simulink model "OFDM_Tx_Rx_fixed_point"  (R2020a)
settings: Solver=FixedStepDiscrete  StartTime=0.0  StopTime=inf  RelTol=1e-3
PostLoadFcn:
  | filter_setup;
InitFcn:
  | % Set parameters
  | fs = 1e6;
  | 
  | % Load all required variables
  | load('read_addr_data');
  | load('read_addr_cp');
  | load('read_addr_pream');
  | load('read_addr_rx');
  | load('pilot');
  | load('sc_index');
  | load('LTSfreq');
  | load('STSfreq');
  | load('LTSread');
  | load('STSread');
values from neighbouring files (symbols this model uses):
  CIC_fine_Rx = 2^(-(CIC_right_shift_Rx-CIC_shift_Rx))    [filter_setup.m]
  CIC_fine_Tx = 2^-(CIC_right_shift - CIC_left_shift - CIC_shift_Tx)    [filter_setup.m]
  STSfreq = [0 0 0 0 0 0 0 0 1 0 0 0 ... (64 elements, 1x64)]    [STSfreq.mat]
undefined symbols (not defined in the file or in its folder): LTSfreq, LTSread, pilot, read_addr_cp, read_addr_data, read_addr_pream, read_addr_rx, sc_index, STSread
libraries: hdlsllib x56, simulink x55, dspmlti4 x8, commseqgen3 x7, dsphdlmathfun x3, dsphdlxfrm x2, dspobslib x1, dsphdlsigops x1
(part 4 of 4)

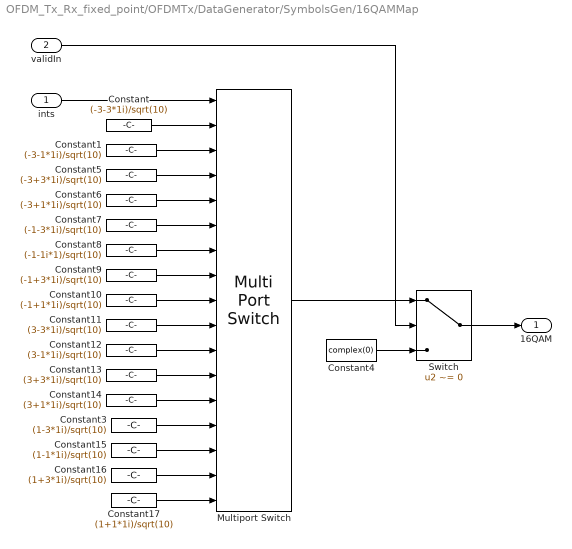
== system OFDM_Tx_Rx_fixed_point/OFDMTx/DataGenerator/SymbolsGen/16QAMMap ==
  ints : Inport
  validIn : Inport  Port=2
  Constant : Constant  Value=(-3-3*1i)/sqrt(10)  VectorParams1D=off  OutDataTypeStr=fixdt(1,16,14)  SampleTime=1/fs
  Constant1 : Constant  Value=(-3-1*1i)/sqrt(10)  VectorParams1D=off  OutDataTypeStr=fixdt(1,16,14)  SampleTime=1/fs
  Constant10 : Constant  Value=(-1+1*1i)/sqrt(10)  VectorParams1D=off  OutDataTypeStr=fixdt(1,16,14)  SampleTime=1/fs
  Constant11 : Constant  Value=(3-3*1i)/sqrt(10)  VectorParams1D=off  OutDataTypeStr=fixdt(1,16,14)  SampleTime=1/fs
  Constant12 : Constant  Value=(3-1*1i)/sqrt(10)  VectorParams1D=off  OutDataTypeStr=fixdt(1,16,14)  SampleTime=1/fs
  Constant13 : Constant  Value=(3+3*1i)/sqrt(10)  VectorParams1D=off  OutDataTypeStr=fixdt(1,16,14)  SampleTime=1/fs
  Constant14 : Constant  Value=(3+1*1i)/sqrt(10)  VectorParams1D=off  OutDataTypeStr=fixdt(1,16,14)  SampleTime=1/fs
  Constant15 : Constant  Value=(1-1*1i)/sqrt(10)  VectorParams1D=off  OutDataTypeStr=fixdt(1,16,14)  SampleTime=1/fs
  Constant16 : Constant  Value=(1+3*1i)/sqrt(10)  VectorParams1D=off  OutDataTypeStr=fixdt(1,16,14)  SampleTime=1/fs
  Constant17 : Constant  Value=(1+1*1i)/sqrt(10)  VectorParams1D=off  OutDataTypeStr=fixdt(1,16,14)  SampleTime=1/fs
  Constant3 : Constant  Value=(1-3*1i)/sqrt(10)  VectorParams1D=off  OutDataTypeStr=fixdt(1,16,14)  SampleTime=1/fs
  Constant4 : Constant  Value=complex(0)  VectorParams1D=off  OutDataTypeStr=fixdt(1,16,14)  SampleTime=1/fs
  Constant5 : Constant  Value=(-3+3*1i)/sqrt(10)  VectorParams1D=off  OutDataTypeStr=fixdt(1,16,14)  SampleTime=1/fs
  Constant6 : Constant  Value=(-3+1*1i)/sqrt(10)  VectorParams1D=off  OutDataTypeStr=fixdt(1,16,14)  SampleTime=1/fs
  Constant7 : Constant  Value=(-1-3*1i)/sqrt(10)  VectorParams1D=off  OutDataTypeStr=fixdt(1,16,14)  SampleTime=1/fs
  Constant8 : Constant  Value=(-1-1i*1)/sqrt(10)  VectorParams1D=off  OutDataTypeStr=fixdt(1,16,14)  SampleTime=1/fs
  Constant9 : Constant  Value=(-1+3*1i)/sqrt(10)  VectorParams1D=off  OutDataTypeStr=fixdt(1,16,14)  SampleTime=1/fs
  Multiport Switch : MultiPortSwitch  DataPortOrder=Zero-based contiguous  Inputs=16  zeroidx=on
  Switch : Switch  Criteria=u2 ~= 0
  16QAM : Outport  VectorParamsAs1DForOutWhenUnconnected=off
  wires:
  Switch/1 -> 16QAM/1
  Constant4/1 -> Switch/3
  Multiport Switch/1 -> Switch/1
  validIn/1 -> Switch/2
  ints/1 -> Multiport Switch/1
  Constant/1 -> Multiport Switch/2
  Constant1/1 -> Multiport Switch/3
  Constant5/1 -> Multiport Switch/4
  Constant6/1 -> Multiport Switch/5
  Constant7/1 -> Multiport Switch/6
  Constant8/1 -> Multiport Switch/7
  Constant9/1 -> Multiport Switch/8
  Constant10/1 -> Multiport Switch/9
  Constant11/1 -> Multiport Switch/10
  Constant12/1 -> Multiport Switch/11
  Constant13/1 -> Multiport Switch/12
  Constant14/1 -> Multiport Switch/13
  Constant3/1 -> Multiport Switch/14
  Constant15/1 -> Multiport Switch/15
  Constant16/1 -> Multiport Switch/16
  Constant17/1 -> Multiport Switch/17

== system OFDM_Tx_Rx_fixed_point/OFDMTx/DataGenerator/SymbolsGen/BPSKmap ==
  bits : Inport
  validIn : Inport  Port=2
  Constant : Constant  Value=complex(-1+0*1i)  VectorParams1D=off  OutDataTypeStr=fixdt(1,16,14)  SampleTime=1/fs
  Constant1 : Constant  Value=complex(1+0*1i)  VectorParams1D=off  OutDataTypeStr=fixdt(1,16,14)  SampleTime=1/fs
  Constant4 : Constant  Value=complex(0)  VectorParams1D=off  OutDataTypeStr=fixdt(1,16,14)  SampleTime=1/fs
  Multiport Switch : MultiPortSwitch  DataPortOrder=Zero-based contiguous  Inputs=2  zeroidx=on
  Switch : Switch  Criteria=u2 ~= 0
  BPSKOut : Outport  VectorParamsAs1DForOutWhenUnconnected=off
  wires:
  Switch/1 -> BPSKOut/1
  Constant4/1 -> Switch/3
  Multiport Switch/1 -> Switch/1
  validIn/1 -> Switch/2
  Constant1/1 -> Multiport Switch/3
  Constant/1 -> Multiport Switch/2
  bits/1 -> Multiport Switch/1

== system OFDM_Tx_Rx_fixed_point/OFDMTx/DataGenerator/SymbolsGen/DataGen16QAM ==
  Bit Concat1 : hdlsllib/Logic and Bit Operations/Bit Concat  numInputs=4
  PN Sequence Generator3 : commseqgen3/PN Sequence Generator  poly='z^6 + z + 1'  ini_sta=[0 0 0 0 0 1]  outBitMaskSource=Dialog parameter  shift=0  outVarSiz=off  maxOutSizeMode=Dialog parameter  maxOutSize=[10 1]  Ts=1/fs  sampPerFrame=1  reset=off  bitPackedOutputs=off  outDataType=boolean  numPackedBits=8  bitPackDataSigned=off  bitPackedOutDType=double
  PN Sequence Generator4 : commseqgen3/PN Sequence Generator  poly='z^6 + z + 1'  ini_sta=[0 0 0 0 1 1]  outBitMaskSource=Dialog parameter  shift=0  outVarSiz=off  maxOutSizeMode=Dialog parameter  maxOutSize=[10 1]  Ts=1/fs  sampPerFrame=1  reset=off  bitPackedOutputs=off  outDataType=boolean  numPackedBits=8  bitPackDataSigned=off  bitPackedOutDType=double
  PN Sequence Generator5 : commseqgen3/PN Sequence Generator  poly='z^6 + z + 1'  ini_sta=[0 0 1 0 1 1]  outBitMaskSource=Dialog parameter  shift=0  outVarSiz=off  maxOutSizeMode=Dialog parameter  maxOutSize=[10 1]  Ts=1/fs  sampPerFrame=1  reset=off  bitPackedOutputs=off  outDataType=boolean  numPackedBits=8  bitPackDataSigned=off  bitPackedOutDType=double
  PN Sequence Generator6 : commseqgen3/PN Sequence Generator  poly='z^6 + z + 1'  ini_sta=[1 0 1 0 1 1]  outBitMaskSource=Dialog parameter  shift=0  outVarSiz=off  maxOutSizeMode=Dialog parameter  maxOutSize=[10 1]  Ts=1/fs  sampPerFrame=1  reset=off  bitPackedOutputs=off  outDataType=boolean  numPackedBits=8  bitPackDataSigned=off  bitPackedOutDType=double
  y : Outport
  wires:
  PN Sequence Generator5/1 -> Bit Concat1/3
  PN Sequence Generator4/1 -> Bit Concat1/2
  PN Sequence Generator6/1 -> Bit Concat1/4
  PN Sequence Generator3/1 -> Bit Concat1/1
  Bit Concat1/1 -> y/1

== system OFDM_Tx_Rx_fixed_point/OFDMTx/DataGenerator/SymbolsGen/DataGenBPSK ==
  PN Sequence Generator : commseqgen3/PN Sequence Generator  poly='z^6 + z + 1'  ini_sta=[0 0 0 0 0 1]  outBitMaskSource=Dialog parameter  shift=0  outVarSiz=off  maxOutSizeMode=Dialog parameter  maxOutSize=[10 1]  Ts=1/fs  sampPerFrame=1  reset=off  bitPackedOutputs=off  outDataType=boolean  numPackedBits=8  bitPackDataSigned=off  bitPackedOutDType=double
  y : Outport
  wires:
  PN Sequence Generator/1 -> y/1

== system OFDM_Tx_Rx_fixed_point/OFDMTx/DataGenerator/SymbolsGen/DataGenQPSK ==
  Bit Concat : hdlsllib/Logic and Bit Operations/Bit Concat  numInputs=2
  PN Sequence Generator1 : commseqgen3/PN Sequence Generator  poly='z^6 + z + 1'  ini_sta=[0 0 0 0 0 1]  outBitMaskSource=Dialog parameter  shift=0  outVarSiz=off  maxOutSizeMode=Dialog parameter  maxOutSize=[10 1]  Ts=1/fs  sampPerFrame=1  reset=off  bitPackedOutputs=off  outDataType=boolean  numPackedBits=8  bitPackDataSigned=off  bitPackedOutDType=double
  PN Sequence Generator2 : commseqgen3/PN Sequence Generator  poly='z^6 + z + 1'  ini_sta=[0 0 0 0 1 1]  outBitMaskSource=Dialog parameter  shift=0  outVarSiz=off  maxOutSizeMode=Dialog parameter  maxOutSize=[10 1]  Ts=1/fs  sampPerFrame=1  reset=off  bitPackedOutputs=off  outDataType=boolean  numPackedBits=8  bitPackDataSigned=off  bitPackedOutDType=double
  y : Outport
  wires:
  Bit Concat/1 -> y/1
  PN Sequence Generator2/1 -> Bit Concat/2
  PN Sequence Generator1/1 -> Bit Concat/1

== system OFDM_Tx_Rx_fixed_point/OFDMTx/DataGenerator/SymbolsGen/QPSKMap ==
  ints : Inport
  validIn : Inport  Port=2
  Constant : Constant  Value=1/sqrt(2) + 1/sqrt(2)*1i  VectorParams1D=off  OutDataTypeStr=fixdt(1,16,14)  SampleTime=1/fs
  Constant1 : Constant  Value=1/sqrt(2) - 1/sqrt(2)*1i  VectorParams1D=off  OutDataTypeStr=fixdt(1,16,14)  SampleTime=1/fs
  Constant2 : Constant  Value=-1/sqrt(2) + 1/sqrt(2)*1i  VectorParams1D=off  OutDataTypeStr=fixdt(1,16,14)  SampleTime=1/fs
  Constant3 : Constant  Value=-1/sqrt(2) - 1/sqrt(2)*1i  VectorParams1D=off  OutDataTypeStr=fixdt(1,16,14)  SampleTime=1/fs
  Constant4 : Constant  Value=complex(0)  VectorParams1D=off  OutDataTypeStr=fixdt(1,16,14)  SampleTime=1/fs
  Multiport Switch : MultiPortSwitch  DataPortOrder=Zero-based contiguous  Inputs=4  zeroidx=on
  Switch : Switch  Criteria=u2 ~= 0
  QPSKOut : Outport  VectorParamsAs1DForOutWhenUnconnected=off
  wires:
  Constant3/1 -> Multiport Switch/5
  Constant2/1 -> Multiport Switch/4
  ints/1 -> Multiport Switch/1
  Constant/1 -> Multiport Switch/2
  Constant1/1 -> Multiport Switch/3
  validIn/1 -> Switch/2
  Multiport Switch/1 -> Switch/1
  Constant4/1 -> Switch/3
  Switch/1 -> QPSKOut/1

== system OFDM_Tx_Rx_fixed_point/OFDMTx/IFFT/IFFTValid/dataIFFTValid ==
  dataValidIn : Inport
  Compare To Constant : simulink/Logic and Bit Operations/Compare To Constant  relop=>=  const=17  OutDataTypeStr=boolean
  Logical Operator : Logic  Operator=NOT  IconShape=distinctive  AllPortsSameDT=off  OutDataTypeStr=boolean
  SAMPLE_COUNTER : hdlsllib/Sources/HDL Counter  CountType=Count limited  CountInit=1  CountStep=1  CountMax=80  CountFromType=Initial value  CountFrom=1  CountResetPort=on  CountLoadPort=off  CountEnbPort=on  CountDirPort=off  CountDataType=Unsigned  CountWordLen=7  CountFracLen=0  CountSampTime=1
  dataIFFTValidOut : Outport  VectorParamsAs1DForOutWhenUnconnected=off
  wires:
  dataValidIn/1 -> SAMPLE_COUNTER/2, Logical Operator/1
  Compare To Constant/1 -> dataIFFTValidOut/1
  Logical Operator/1 -> SAMPLE_COUNTER/1
  SAMPLE_COUNTER/1 -> Compare To Constant/1

== system OFDM_Tx_Rx_fixed_point/OFDMTx/IFFT/IFFTValid/preambIFFTValid ==
  preambValid : Inport
  AND{,1..3} (4 alike) : Logic  IconShape=distinctive  AllPortsSameDT=off  OutDataTypeStr=boolean
  Compare To Constant1 : simulink/Logic and Bit Operations/Compare To Constant  relop=>=  const=96  OutDataTypeStr=boolean
  Compare To Constant2 : simulink/Logic and Bit Operations/Compare To Constant  relop=<=  const=159  OutDataTypeStr=boolean
  Compare To Constant3 : simulink/Logic and Bit Operations/Compare To Constant  relop=>=  const=256  OutDataTypeStr=boolean
  Compare To Constant4 : simulink/Logic and Bit Operations/Compare To Constant  relop=<=  const=319  OutDataTypeStr=boolean
  HDL Counter1 : hdlsllib/Sources/HDL Counter  CountType=Count limited  CountInit=0  CountStep=1  CountMax=319  CountFromType=Initial value  CountFrom=0  CountResetPort=on  CountLoadPort=off  CountEnbPort=on  CountDirPort=off  CountDataType=Unsigned  CountWordLen=9  CountFracLen=0  CountSampTime=1
  NOT : Logic  Operator=NOT  IconShape=distinctive  AllPortsSameDT=off  OutDataTypeStr=boolean
  OR : Logic  Operator=OR  IconShape=distinctive  AllPortsSameDT=off  OutDataTypeStr=boolean
  preambIFFTValidOut : Outport  VectorParamsAs1DForOutWhenUnconnected=off
  wires:
  AND/1 -> AND1/1
  AND2/1 -> AND3/1
  HDL Counter1/1 -> Compare To Constant4/1, Compare To Constant3/1, Compare To Constant2/1, Compare To Constant1/1
  OR/1 -> preambIFFTValidOut/1
  preambValid/1 -> HDL Counter1/2, AND3/2, AND1/2, NOT/1
  Compare To Constant1/1 -> AND/1
  Compare To Constant4/1 -> AND2/2
  AND1/1 -> OR/1
  AND3/1 -> OR/2
  Compare To Constant2/1 -> AND/2
  NOT/1 -> HDL Counter1/1
  Compare To Constant3/1 -> AND2/1

== system OFDM_Tx_Rx_fixed_point/OFDMTx/SCMapper/DataMapper/READ_CTRL2 ==
  In1 : Inport
  In2 : Inport  Port=2
  Constant : Constant  Value=0  OutDataTypeStr=fixdt(0,8,0)  SampleTime=1/fs
  Switch : Switch  Criteria=u2 ~= 0
  Out1 : Outport  VectorParamsAs1DForOutWhenUnconnected=off
  wires:
  Switch/1 -> Out1/1
  In1/1 -> Switch/1
  In2/1 -> Switch/2
  Constant/1 -> Switch/3

== system OFDM_Tx_Rx_fixed_point/OFDMTx/SCMapper/PremableMapper/READ_CTRL ==
  In1 : Inport
  In2 : Inport  Port=2
  Constant : Constant  Value=0  OutDataTypeStr=fixdt(0,8,0)  SampleTime=1/fs
  Switch : Switch  Criteria=u2 ~= 0
  Out1 : Outport  VectorParamsAs1DForOutWhenUnconnected=off
  wires:
  Switch/1 -> Out1/1
  In1/1 -> Switch/1
  In2/1 -> Switch/2
  Constant/1 -> Switch/3

== system OFDM_Tx_Rx_fixed_point/OFDMRx/PhaseTracking_1/PilotCtrlGen/pilotGen/ToComplex1 ==
  In1 : Inport
  Constant1 : Constant  Value=0  OutDataTypeStr=fixdt(1,2,0)  SampleTime=1/fs
  Real-Imag to Complex : RealImagToComplex
  Out1 : Outport  VectorParamsAs1DForOutWhenUnconnected=off
  wires:
  Real-Imag to Complex/1 -> Out1/1
  In1/1 -> Real-Imag to Complex/1
  Constant1/1 -> Real-Imag to Complex/2

== system OFDM_Tx_Rx_fixed_point/OFDMRx/PhaseTracking_2/PilotCtrlGen/pilotGen/ToComplex1 ==
  In1 : Inport
  Constant1 : Constant  Value=0  OutDataTypeStr=fixdt(1,2,0)  SampleTime=1/fs
  Real-Imag to Complex : RealImagToComplex
  Out1 : Outport  VectorParamsAs1DForOutWhenUnconnected=off
  wires:
  Real-Imag to Complex/1 -> Out1/1
  In1/1 -> Real-Imag to Complex/1
  Constant1/1 -> Real-Imag to Complex/2

== system OFDM_Tx_Rx_fixed_point/OFDMRx/Synchronisation/ControlSigGen/PreambleValidGen/RisingEdge ==
  ValidIn : Inport
  Delay : Delay  DelayLength=1
  Relational Operator : RelationalOperator  Operator=>  OutDataTypeStr=boolean  RndMeth=Nearest
  Out1 : Outport
  wires:
  Relational Operator/1 -> Out1/1
  Delay/1 -> Relational Operator/2
  ValidIn/1 -> Delay/1, Relational Operator/1

== matlab function OFDM_Tx_Rx_fixed_point/OFDMTx/DataGenerator/Data Multiplexer ==
  data: symbols input; dataready input; data output; pilots input; pval input; sts input; stsval input; lts input; ltsval input
function data  = dataMux(symbols,dataready,pilots,pval,sts,stsval,lts,ltsval)
% Data multiplexer 
if (pval == true)
    data = pilots; 
elseif (stsval == true)
    data = sts; 
elseif (ltsval == true)
    data = lts; 
elseif (dataready == true) 
    data = symbols;
else 
    data = fi(complex(0),1,16,14);
end

== matlab function OFDM_Tx_Rx_fixed_point/OFDMRx/PhaseTracking_1/CordicRotate/QCORR/QUAD_MAP1 ==
  data: xin input; xout output; yout output; yin input; ctrl input
function [xout,yout] = fcn(xin,yin,ctrl)
% Process to perform final rotation 
% by pi/2 if the original angle was 
% in 3rd or 4th quadrants    
if ctrl == 0
    % 1st or 2nd quadrants 
    xout = fi(xin,1,21,15);  
    yout = fi(yin,1,21,15);  
elseif ctrl == 1
    % 3rd quadrant (rotate pi/2 clockwise)
    xout = fi(yin,1,21,15); 
    yout = fi(-xin,1,21,15); 
elseif ctrl == 2
    % 4th quadrant (rotate pi/2 anti-clockwise) 
    xout = fi(-yin,1,21,15); 
    yout = fi(xin,1,21,15); 
else 
    % others clause
    xout = fi(xin,1,21,15); 
    yout = fi(yin,1,21,15); 
end

== matlab function OFDM_Tx_Rx_fixed_point/OFDMTx/SCMapper/Mux2 ==
  data: preamb input; preambVal input; dataOut output; data input; dataVal input
function dataOut = mux(preamb,preambVal,data,dataVal)

if (preambVal == true)
    dataOut = preamb; 
elseif (dataVal == true)
    dataOut = data; 
else 
    dataOut = fi(complex(0),1,16,14);
end

== matlab function OFDM_Tx_Rx_fixed_point/OFDMTx/CPAdd/Mux2 ==
  data: sts input; stsval input; lts input; ltsval input; dataOut output; data input; dataval input
function dataOut = mux(sts,stsval,lts,ltsval,data,dataval)

if (stsval == true)
    dataOut = sts; 
elseif (ltsval == true)
    dataOut = lts; 
elseif (dataval == true) 
    dataOut = data; 
else 
    dataOut = fi(complex(0),1,16,14);
end

== matlab function OFDM_Tx_Rx_fixed_point/OFDMRx/PhaseTracking_1/CordicRotate/QUAD_MAP/QUAD_DETERM1 ==
  data: ang_in input; ang_out output; QUAD output
function [ang_out,QUAD] = fcn(ang_in)
% Process to determine quadrant and 
% shift into region -pi/2 to pi/2 if 
% not already there 
v = fi(pi,1,23,20);
x = fi(-pi,1,23,20); 
y = fi(-pi/2,1,23,20); 
z = fi(pi/2,1,23,20);

% Determine quadrant 
if ((ang_in >= y) && (ang_in <= z))
    QUAD = fi(0,0,2,0); % Quads 1 or 2
elseif ((ang_in < y) && (ang_in >= x))
    QUAD = fi(1,0,2,0); % Quad 3
elseif ((ang_in > z) && (ang_in <= v))
    QUAD = fi(2,0,2,0); % Quad 4
else 
    % others clause
    QUAD = fi(0,0,2,0);
end 

% Determine whether we need to add or subtract pi/2 
% based on quadrant location
switch(QUAD) 
    
    case 0 
        % Angle stays the same 
        ang_out = fi(ang_in, 1, 23, 20); 
    case 1
        % pi/2 is added to angle (anti-clockwise)
        ang_out = fi(ang_in + z, 1, 23, 20); 
    case 2
        % pi/2 is subtracted from angle (clockwise)
        ang_out = fi(ang_in - z, 1, 23, 20); 
    otherwise
        % others clause make output angle 
        % equal to input angle  
        ang_out = fi(ang_in, 1, 23, 20); 
end

== matlab function OFDM_Tx_Rx_fixed_point/OFDMRx/PhaseTracking_2/CordicRotate/QCORR/QUAD_MAP1 ==
  data: xin input; xout output; yout output; yin input; ctrl input
function [xout,yout] = fcn(xin,yin,ctrl)
% Process to perform final rotation 
% by pi/2 if the original angle was 
% in 3rd or 4th quadrants    
if ctrl == 0
    % 1st or 2nd quadrants 
    xout = fi(xin,1,21,15);  
    yout = fi(yin,1,21,15);  
elseif ctrl == 1
    % 3rd quadrant (rotate pi/2 clockwise)
    xout = fi(yin,1,21,15); 
    yout = fi(-xin,1,21,15); 
elseif ctrl == 2
    % 4th quadrant (rotate pi/2 anti-clockwise) 
    xout = fi(-yin,1,21,15); 
    yout = fi(xin,1,21,15); 
else 
    % others clause
    xout = fi(xin,1,21,15); 
    yout = fi(yin,1,21,15); 
end

== matlab function OFDM_Tx_Rx_fixed_point/OFDMRx/PhaseTracking_2/CordicRotate/QUAD_MAP/QUAD_DETERM1 ==
  data: ang_in input; ang_out output; QUAD output
function [ang_out,QUAD] = fcn(ang_in)
% Process to determine quadrant and 
% shift into region -pi/2 to pi/2 if 
% not already there 
v = fi(pi,1,23,20);
x = fi(-pi,1,23,20); 
y = fi(-pi/2,1,23,20); 
z = fi(pi/2,1,23,20);

% Determine quadrant 
if ((ang_in >= y) && (ang_in <= z))
    QUAD = fi(0,0,2,0); % Quads 1 or 2
elseif ((ang_in < y) && (ang_in >= x))
    QUAD = fi(1,0,2,0); % Quad 3
elseif ((ang_in > z) && (ang_in <= v))
    QUAD = fi(2,0,2,0); % Quad 4
else 
    % others clause
    QUAD = fi(0,0,2,0);
end 

% Determine whether we need to add or subtract pi/2 
% based on quadrant location
switch(QUAD) 
    
    case 0 
        % Angle stays the same 
        ang_out = fi(ang_in, 1, 23, 20); 
    case 1
        % pi/2 is added to angle (anti-clockwise)
        ang_out = fi(ang_in + z, 1, 23, 20); 
    case 2
        % pi/2 is subtracted from angle (clockwise)
        ang_out = fi(ang_in - z, 1, 23, 20); 
    otherwise
        % others clause make output angle 
        % equal to input angle  
        ang_out = fi(ang_in, 1, 23, 20); 
end
